simulink model "AT_and_specifications_breach"  (R2019b)
settings: Solver=FixedStepAuto  StartTime=0.0  StopTime=tspan(end)  FixedStep=fixedStepSize  RelTol=1e-3
settings Model: Creator=JEDDELAN  LastModifiedBy=JEDDELAN
settings DataIOCC: ExternalInput=[t__, u__]  LoadExternalInput=on  SaveFormat=StructureWithTime
settings DebuggingCC: ArithmeticOperatorsInVariantConditions=warning
settings SFSimCC: SimUseLocalCustomCode=off  CustomCodeUndefinedFunction=UseInterfaceOnly
settings RTWCC: RTWUseLocalCustomCode=off

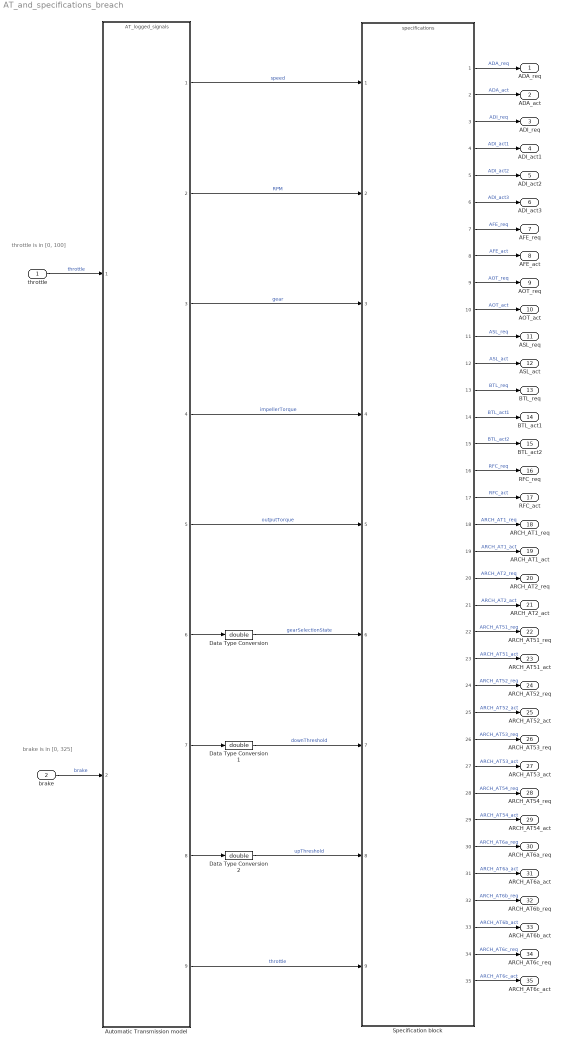
== system AT_and_specifications_breach ==
  note: throttle is in [0, 100]
  note: brake is in [0, 325]
  throttle : Inport
  brake : Inport  Port=2
  Automatic Transmission model : ModelReference  ModelNameDialog=AT_logged_signals.mdl  SimulationMode=Normal  ModelReferenceVersion=1.276
  Data Type Conversion : DataTypeConversion  OutDataTypeStr=double
  Data Type Conversion1 : DataTypeConversion  OutDataTypeStr=double
  Data Type Conversion2 : DataTypeConversion  OutDataTypeStr=double
  Specification block : ModelReference  ModelNameDialog=specifications  SimulationMode=Normal  ModelReferenceVersion=1.32
  ADA_req : Outport  VectorParamsAs1DForOutWhenUnconnected=off
  ADA_act : Outport  Port=2  VectorParamsAs1DForOutWhenUnconnected=off
  ADI_req : Outport  Port=3  VectorParamsAs1DForOutWhenUnconnected=off
  ADI_act1 : Outport  Port=4  VectorParamsAs1DForOutWhenUnconnected=off
  ADI_act2 : Outport  Port=5  VectorParamsAs1DForOutWhenUnconnected=off
  ADI_act3 : Outport  Port=6  VectorParamsAs1DForOutWhenUnconnected=off
  AFE_req : Outport  Port=7  VectorParamsAs1DForOutWhenUnconnected=off
  AFE_act : Outport  Port=8  VectorParamsAs1DForOutWhenUnconnected=off
  AOT_req : Outport  Port=9  VectorParamsAs1DForOutWhenUnconnected=off
  AOT_act : Outport  Port=10  VectorParamsAs1DForOutWhenUnconnected=off
  ASL_req : Outport  Port=11  VectorParamsAs1DForOutWhenUnconnected=off
  ASL_act : Outport  Port=12  VectorParamsAs1DForOutWhenUnconnected=off
  BTL_req : Outport  Port=13  VectorParamsAs1DForOutWhenUnconnected=off
  BTL_act1 : Outport  Port=14  VectorParamsAs1DForOutWhenUnconnected=off
  BTL_act2 : Outport  Port=15  VectorParamsAs1DForOutWhenUnconnected=off
  RFC_req : Outport  Port=16  VectorParamsAs1DForOutWhenUnconnected=off
  RFC_act : Outport  Port=17  VectorParamsAs1DForOutWhenUnconnected=off
  ARCH_AT1_req : Outport  Port=18  VectorParamsAs1DForOutWhenUnconnected=off
  ARCH_AT1_act : Outport  Port=19  VectorParamsAs1DForOutWhenUnconnected=off
  ARCH_AT2_req : Outport  Port=20  VectorParamsAs1DForOutWhenUnconnected=off
  ARCH_AT2_act : Outport  Port=21  VectorParamsAs1DForOutWhenUnconnected=off
  ARCH_AT51_req : Outport  Port=22  VectorParamsAs1DForOutWhenUnconnected=off
  ARCH_AT51_act : Outport  Port=23  VectorParamsAs1DForOutWhenUnconnected=off
  ARCH_AT52_req : Outport  Port=24  VectorParamsAs1DForOutWhenUnconnected=off
  ARCH_AT52_act : Outport  Port=25  VectorParamsAs1DForOutWhenUnconnected=off
  ARCH_AT53_req : Outport  Port=26  VectorParamsAs1DForOutWhenUnconnected=off
  ARCH_AT53_act : Outport  Port=27  VectorParamsAs1DForOutWhenUnconnected=off
  ARCH_AT54_req : Outport  Port=28  VectorParamsAs1DForOutWhenUnconnected=off
  ARCH_AT54_act : Outport  Port=29  VectorParamsAs1DForOutWhenUnconnected=off
  ARCH_AT6a_req : Outport  Port=30  VectorParamsAs1DForOutWhenUnconnected=off
  ARCH_AT6a_act : Outport  Port=31  VectorParamsAs1DForOutWhenUnconnected=off
  ARCH_AT6b_req : Outport  Port=32  VectorParamsAs1DForOutWhenUnconnected=off
  ARCH_AT6b_act : Outport  Port=33  VectorParamsAs1DForOutWhenUnconnected=off
  ARCH_AT6c_req : Outport  Port=34  VectorParamsAs1DForOutWhenUnconnected=off
  ARCH_AT6c_act : Outport  Port=35  VectorParamsAs1DForOutWhenUnconnected=off
  wires:
  throttle/1 -> Automatic Transmission model/1  "throttle"
  brake/1 -> Automatic Transmission model/2  "brake"
  Specification block/1 -> ADA_req/1  "ADA_req"
  Specification block/2 -> ADA_act/1  "ADA_act"
  Specification block/3 -> ADI_req/1  "ADI_req"
  Specification block/4 -> ADI_act1/1  "ADI_act1"
  Specification block/5 -> ADI_act2/1  "ADI_act2"
  Specification block/6 -> ADI_act3/1  "ADI_act3"
  Specification block/7 -> AFE_req/1  "AFE_req"
  Specification block/8 -> AFE_act/1  "AFE_act"
  Automatic Transmission model/1 -> Specification block/1  "speed"
  Automatic Transmission model/2 -> Specification block/2  "RPM"
  Automatic Transmission model/3 -> Specification block/3  "gear"
  Automatic Transmission model/4 -> Specification block/4  "impellerTorque"
  Automatic Transmission model/5 -> Specification block/5  "outputTorque"
  Automatic Transmission model/6 -> Data Type Conversion/1
  Automatic Transmission model/7 -> Data Type Conversion1/1
  Automatic Transmission model/8 -> Data Type Conversion2/1
  Automatic Transmission model/9 -> Specification block/9  "throttle"
  Data Type Conversion/1 -> Specification block/6  "gearSelectionState"
  Specification block/9 -> AOT_req/1  "AOT_req"
  Specification block/10 -> AOT_act/1  "AOT_act"
  Specification block/11 -> ASL_req/1  "ASL_req"
  Specification block/12 -> ASL_act/1  "ASL_act"
  Specification block/13 -> BTL_req/1  "BTL_req"
  Specification block/14 -> BTL_act1/1  "BTL_act1"
  Data Type Conversion1/1 -> Specification block/7  "downThreshold"
  Data Type Conversion2/1 -> Specification block/8  "upThreshold"
  Specification block/15 -> BTL_act2/1  "BTL_act2"
  Specification block/16 -> RFC_req/1  "RFC_req"
  Specification block/17 -> RFC_act/1  "RFC_act"
  Specification block/18 -> ARCH_AT1_req/1  "ARCH_AT1_req"
  Specification block/19 -> ARCH_AT1_act/1  "ARCH_AT1_act"
  Specification block/25 -> ARCH_AT52_act/1  "ARCH_AT52_act"
  Specification block/24 -> ARCH_AT52_req/1  "ARCH_AT52_req"
  Specification block/20 -> ARCH_AT2_req/1  "ARCH_AT2_req"
  Specification block/21 -> ARCH_AT2_act/1  "ARCH_AT2_act"
  Specification block/22 -> ARCH_AT51_req/1  "ARCH_AT51_req"
  Specification block/23 -> ARCH_AT51_act/1  "ARCH_AT51_act"
  Specification block/26 -> ARCH_AT53_req/1  "ARCH_AT53_req"
  Specification block/35 -> ARCH_AT6c_act/1  "ARCH_AT6c_act"
  Specification block/34 -> ARCH_AT6c_req/1  "ARCH_AT6c_req"
  Specification block/33 -> ARCH_AT6b_act/1  "ARCH_AT6b_act"
  Specification block/32 -> ARCH_AT6b_req/1  "ARCH_AT6b_req"
  Specification block/31 -> ARCH_AT6a_act/1  "ARCH_AT6a_act"
  Specification block/30 -> ARCH_AT6a_req/1  "ARCH_AT6a_req"
  Specification block/29 -> ARCH_AT54_act/1  "ARCH_AT54_act"
  Specification block/28 -> ARCH_AT54_req/1  "ARCH_AT54_req"
  Specification block/27 -> ARCH_AT53_act/1  "ARCH_AT53_act"
